simulink model "feedback_linearization_kalman_filter_sim1"  (R2021b)
settings: Solver=VariableStepAuto  StartTime=0.0  StopTime=500  RelTol=1e-3
undefined symbols (not defined in the file): sim_output_sample_time, sim_u
libraries: simulink x1
settings Model: Creator=Alghisi  LastModifiedBy=alefr
settings DataIOCC: ReturnWorkspaceOutputs=off
settings DebuggingCC: UnconnectedInputMsg=none  UnconnectedOutputMsg=none  UnconnectedLineMsg=none
settings RTWCC: DLArmComputeVersion=20.02.1

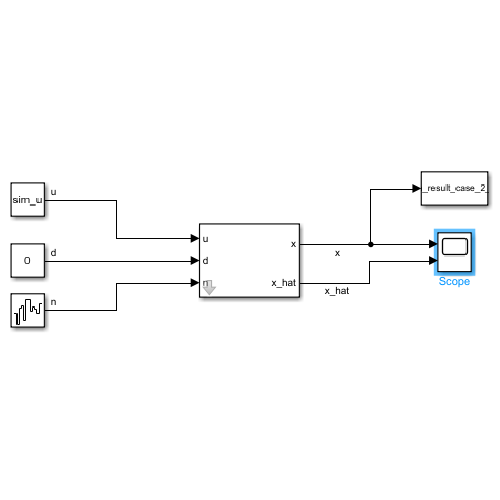
[thumbnail: Simulink's stored preview of the top-level diagram]
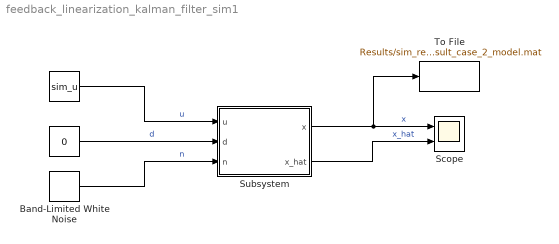
== system feedback_linearization_kalman_filter_sim1 ==
  "  " : Constant  Value=0
  "       " : Constant  Value=sim_u
  Band-Limited White Noise : simulink/Sources/Band-Limited White Noise  Cov=1  Ts=0.1  seed=[23341]
  Scope : Scope  NumInputPorts=2
  Subsystem : Subsystem  mask{init_state_param=[8;8]}
      mask prompts: init_state_param "Initial state"
  To File : ToFile  Filename=Results/sim_result_case_2_model.mat  MatrixName=sim_result_case_2_model  SaveFormat=Timeseries  SampleTime=sim_output_sample_time
  wires:
  "  "/1 -> Subsystem/2(d)  "d"
  Band-Limited White Noise/1 -> Subsystem/3(n)  "n"
  Subsystem/1(x) -> To File/1, Scope/1  "x"
  "       "/1 -> Subsystem/1(u)  "u"
  Subsystem/2(x_hat) -> Scope/2  "x_hat"

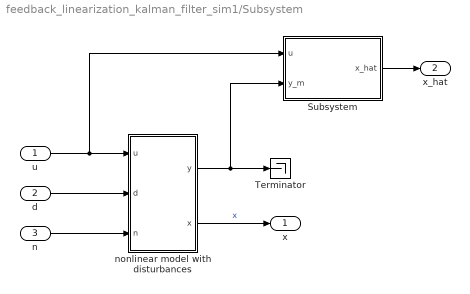
== system feedback_linearization_kalman_filter_sim1/Subsystem ==
  u : Inport
  d : Inport  Port=2
  n : Inport  Port=3
  Subsystem : Subsystem
  Terminator : Terminator
  nonlinear model with disturbances : Subsystem
  x : Outport
  x_hat : Outport  Port=2
  wires:
  n/1 -> nonlinear model with disturbances/3(n)
  u/1 -> Subsystem/1(u), nonlinear model with disturbances/1(u)
  nonlinear model with disturbances/1(y) -> Terminator/1, Subsystem/2(y_m)
  nonlinear model with disturbances/2(x) -> x/1  "x"
  d/1 -> nonlinear model with disturbances/2(d)
  Subsystem/1(x_hat) -> x_hat/1

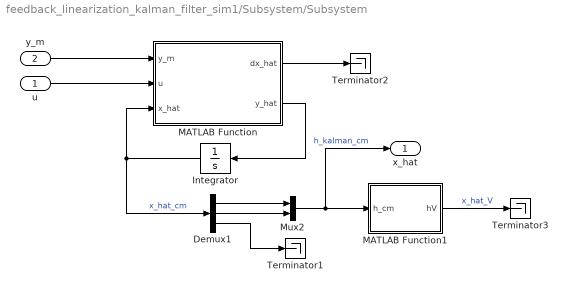
== system feedback_linearization_kalman_filter_sim1/Subsystem/Subsystem ==
  u : Inport
  y_m : Inport  Port=2
  Demux1 : Demux  Outputs=3
  Integrator : Integrator  InitialCondition=[init_state_param;0]
  MATLAB Function : MATLAB Function  TreatAsAtomicUnit=on
  MATLAB Function1 : MATLAB Function  TreatAsAtomicUnit=on
  Mux2 : Mux  Inputs=2
  Terminator1 : Terminator
  Terminator2 : Terminator
  Terminator3 : Terminator
  x_hat : Outport
  wires:
  Demux1/3 -> Terminator1/1
  Mux2/1 -> x_hat/1, MATLAB Function1/1(h_cm)  "h_kalman_cm"
  MATLAB Function/2(y_hat) -> Integrator/1
  Integrator/1 -> MATLAB Function/3(x_hat), Demux1/1  "x_hat_cm"
  Demux1/1 -> Mux2/1
  Demux1/2 -> Mux2/2
  u/1 -> MATLAB Function/2(u)
  MATLAB Function1/1(hV) -> Terminator3/1  "x_hat_V"
  MATLAB Function/1(dx_hat) -> Terminator2/1
  y_m/1 -> MATLAB Function/1(y_m)

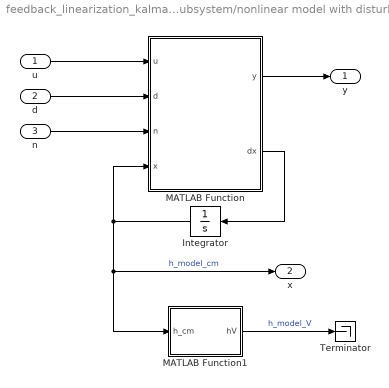
== system feedback_linearization_kalman_filter_sim1/Subsystem/nonlinear model with disturbances ==
  u : Inport
  d : Inport  Port=2
  n : Inport  Port=3
  Integrator : Integrator  InitialCondition=init_state_param
  MATLAB Function : MATLAB Function  TreatAsAtomicUnit=on
  MATLAB Function1 : MATLAB Function  TreatAsAtomicUnit=on
  Terminator : Terminator
  y : Outport
  x : Outport  Port=2
  wires:
  MATLAB Function/1(y) -> y/1
  n/1 -> MATLAB Function/3(n)
  MATLAB Function1/1(hV) -> Terminator/1  "h_model_V"
  d/1 -> MATLAB Function/2(d)
  MATLAB Function/2(dx) -> Integrator/1
  Integrator/1 -> MATLAB Function/4(x), MATLAB Function1/1(h_cm), x/1  "h_model_cm"
  u/1 -> MATLAB Function/1(u)

== matlab function feedback_linearization_kalman_filter_sim1/Subsystem/Subsystem/MATLAB Function1 ==
  data: h_cm input; hV output
function hV = g(h_cm)

hV = h_cm*7.456422751238219e-1 - 1.648066384406454;

== matlab function feedback_linearization_kalman_filter_sim1/Subsystem/Subsystem/MATLAB Function ==
  data: y_m input; u input; x_hat input; dx_hat output; y_hat output
function [dx_hat,y_hat]  = kalman_filter(y_m,u,x_hat)

h1_hat = x_hat(1);
h2_hat = x_hat(2);
w  = x_hat(3);

dx_hat = [h1_hat.*(-3.409145021215564e-2)-h2_hat.*4.707003693403067e-1+u.*2.098905560223643e-1+y_m.*6.312683508484573e-1-sqrt(5.0).*sqrt(7.63e+2).*w.*(4.0./5.5e+1)+9.799223895936294e-1;h1_hat.*3.409145021215564e-2-h2_hat.*1.823621215877478e-1+y_m.*1.988496043239638e-1+3.277173484388491e-1;h2_hat.*7.456422751238219e-3-y_m./1.0e+2-1.648066384406454e-2];

y_hat = h2_hat.*7.456422751238219e-1-1.648066384406454;

== matlab function feedback_linearization_kalman_filter_sim1/Subsystem/nonlinear model with disturbances/MATLAB Function ==
  data: y output; u input; dx output; d input; n input; x input
function [y,dx] = nonlinear_model(u,d,n,x)

x1 = x(1);
x2 = x(2);

y = x2.*7.456422751238219e-1+n-1.648066384406454;

dx = [1+u.*2.818591167129287e-1-(d.*sqrt(x1.*1.962e+3+6.2784e+3))./3.3e+1-sqrt(x1.*1.962e+3+6.2784e+3).*5.151515151515152e-3-u.^2.*2.476601319356684e-2+u.^3.*8.808489605974691e-4+3.751072019731431e-1;sqrt(x1.*1.962e+3+6.2784e+3).*5.151515151515152e-3-sqrt(x2.*1.962e+3+6.2784e+3).*5.151515151515152e-3];

== matlab function feedback_linearization_kalman_filter_sim1/Subsystem/nonlinear model with disturbances/MATLAB Function1 ==
  data: h_cm input; hV output
function hV = g(h_cm)

hV = h_cm*7.456422751238219e-1 - 1.648066384406454;
